simulink model "AMBF"  (R2021a)
settings: Solver=VariableStepAuto  StartTime=0.0  StopTime=10.0  RelTol=1e-3
libraries: robotlib x1
settings Model: Creator=nathanielgoldfarb  LastModifiedBy=nathanielgoldfarb

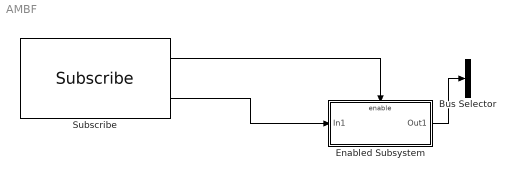
== system AMBF ==
  Bus Selector : BusSelector  OutputSignals=signal1,signal2
  Enabled Subsystem : Subsystem  TreatAsAtomicUnit=on
  Subscribe : robotlib/Subscribe  topicSource=Select from ROS network  topic=/my_topic  messageType=geometry_msgs/Point  SampleTime=-1  legacyBusStruct=off  messageQueueLength=1
  wires:
  Subscribe/1 -> Enabled Subsystem/Enable
  Subscribe/2 -> Enabled Subsystem/1(In1)
  Enabled Subsystem/1(Out1) -> Bus Selector/1

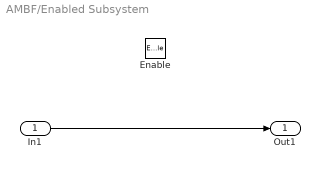
== system AMBF/Enabled Subsystem ==
  In1 : Inport
  Enable : EnablePort
  Out1 : Outport
  wires:
  In1/1 -> Out1/1
